simulink library "Memory_Blocks_Lib"  (R2023a)
settings: Solver=ode45  StartTime=0.0  StopTime=10.0  RelTol=1e-3  EnableMultiTasking=on
libraries: simulink_extras x17
settings Model: Creator=uzivatel  LastModifiedBy=Jozko Mrkvicka
settings SolverCC: AlgebraicLoopSolver=TrustRegion
settings DataIOCC: LimitDataPoints=on  SaveFormat=Array  ReturnWorkspaceOutputs=off
settings OptimizationCC: LifeSpan=inf
settings DebuggingCC: UnderspecifiedInitializationDetection=Classic  MergeDetectMultiDrivingBlocksExec=none  SolverPrmCheckMsg=warning  UnconnectedInputMsg=warning  UnconnectedOutputMsg=warning  UnconnectedLineMsg=warning  StateNameClashWarn=warning  SFUnexpectedBacktrackingDiag=warning  SFNoUnconditionalDefaultTransitionDiag=warning  ArithmeticOperatorsInVariantConditions=warning
settings HardwareCC: ProdBitPerPointer=32  ProdBitPerSizeT=32  ProdBitPerPtrDiffT=32  ProdLargestAtomicFloat=None  ProdIntDivRoundTo=Undefined  ProdEndianess=Unspecified  ProdWordSize=32  ProdHWDeviceType=32-bit Generic
settings ModelReferenceCC: EnableRefExpFcnMdlSchedulingChecks=on  PropagateSignalLabelsOutOfModel=off
settings SFSimCC: SimUseLocalCustomCode=off  CustomCodeUndefinedFunction=UseInterfaceOnly
settings RTWCC: RTWUseLocalCustomCode=off
settings CodeAppCC: StateflowObjectComments=on
settings GRTTargetCC: TargetLangStandard=C89/C90 (ANSI)
settings ConfigComp: CovMetricSettings=dw  CovSaveCumulativeToWorkspaceVar=on  CovSaveSingleToWorkspaceVar=on  CovExternalEMLEnable=off

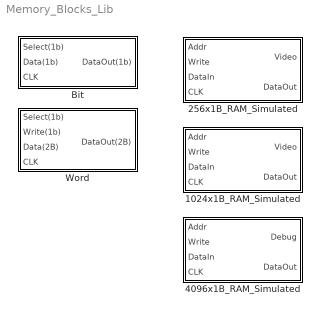
== system Memory_Blocks_Lib ==
  1024x1B_RAM_Simulated : MATLAB Function  TreatAsAtomicUnit=on
  256x1B_RAM_Simulated : MATLAB Function  TreatAsAtomicUnit=on
  4096x1B_RAM_Simulated : MATLAB Function  TreatAsAtomicUnit=on
  Bit : Subsystem
  Word : Subsystem

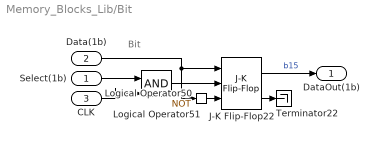
== system Memory_Blocks_Lib/Bit ==
  note: Bit
  Select(1b) : Inport  OutDataTypeStr=boolean
  Data(1b) : Inport  Port=2  OutDataTypeStr=boolean
  CLK : Inport  Port=3  OutDataTypeStr=double
  J-K Flip-Flop22 : simulink_extras/Flip Flops/J-K Flip-Flop  initial_condition=0
  Logical Operator50 : Logic  Operator=NOT  IconShape=distinctive  AllPortsSameDT=off  OutDataTypeStr=boolean
  Logical Operator51 : Logic  IconShape=distinctive  AllPortsSameDT=off  OutDataTypeStr=boolean
  Terminator22 : Terminator
  DataOut(1b) : Outport
  wires:
  Select(1b)/1 -> Logical Operator51/1
  Logical Operator50/1 -> J-K Flip-Flop22/3
  CLK/1 -> Logical Operator51/2
  Data(1b)/1 -> Logical Operator50/1, J-K Flip-Flop22/1
  J-K Flip-Flop22/2 -> Terminator22/1
  J-K Flip-Flop22/1 -> DataOut(1b)/1  "b15"
  Logical Operator51/1 -> J-K Flip-Flop22/2

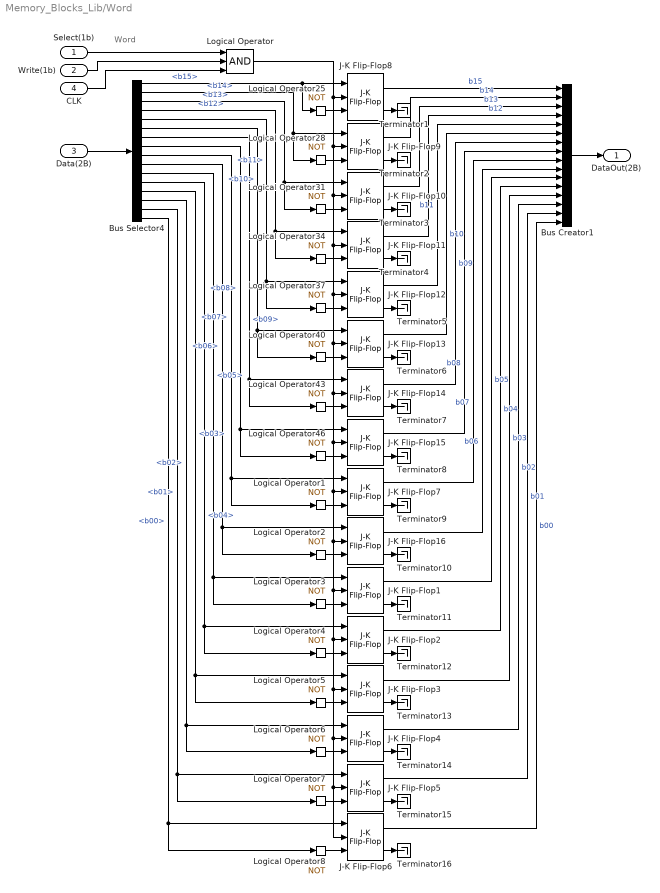
== system Memory_Blocks_Lib/Word ==
  note: Word
  Select(1b) : Inport
  Write(1b) : Inport  Port=2
  Data(2B) : Inport  Port=3
  CLK : Inport  Port=4
  Bus Creator1 : BusCreator  Inputs=16
  Bus Selector4 : BusSelector  OutputSignals=b15,b14,b13,b12,b11,b10,b09,b08,b07,b06,b05,b04,b03,b02,b01,b00
  J-K Flip-Flop{1..16} (16 alike) : simulink_extras/Flip Flops/J-K Flip-Flop  initial_condition=0
  Logical Operator : Logic  Inputs=3  IconShape=distinctive  AllPortsSameDT=off  OutDataTypeStr=boolean
  Logical Operator{1..8,25,28,31,34,37,40,43,46} (16 alike) : Logic  Operator=NOT  IconShape=distinctive  AllPortsSameDT=off  OutDataTypeStr=boolean
  Terminator{1..16} (16 alike) : Terminator
  DataOut(2B) : Outport
  wires:
  Write(1b)/1 -> Logical Operator/2
  Data(2B)/1 -> Bus Selector4/1
  Logical Operator25/1 -> J-K Flip-Flop8/3
  J-K Flip-Flop8/1 -> Bus Creator1/1  "b15"
  J-K Flip-Flop8/2 -> Terminator1/1
  Logical Operator28/1 -> J-K Flip-Flop9/3
  J-K Flip-Flop9/1 -> Bus Creator1/2  "b14"
  J-K Flip-Flop9/2 -> Terminator2/1
  Bus Selector4/2 -> Logical Operator28/1, J-K Flip-Flop9/1  "<b14>"
  Logical Operator31/1 -> J-K Flip-Flop10/3
  J-K Flip-Flop10/1 -> Bus Creator1/3  "b13"
  J-K Flip-Flop10/2 -> Terminator3/1
  Bus Selector4/3 -> Logical Operator31/1, J-K Flip-Flop10/1  "<b13>"
  Logical Operator34/1 -> J-K Flip-Flop11/3
  J-K Flip-Flop11/1 -> Bus Creator1/4  "b12"
  J-K Flip-Flop11/2 -> Terminator4/1
  Bus Selector4/4 -> J-K Flip-Flop11/1, Logical Operator34/1  "<b12>"
  Logical Operator37/1 -> J-K Flip-Flop12/3
  J-K Flip-Flop12/1 -> Bus Creator1/5  "b11"
  J-K Flip-Flop12/2 -> Terminator5/1
  Bus Selector4/5 -> J-K Flip-Flop12/1, Logical Operator37/1  "<b11>"
  Logical Operator40/1 -> J-K Flip-Flop13/3
  J-K Flip-Flop13/1 -> Bus Creator1/6  "b10"
  J-K Flip-Flop13/2 -> Terminator6/1
  Bus Selector4/6 -> J-K Flip-Flop13/1, Logical Operator40/1  "<b10>"
  Logical Operator43/1 -> J-K Flip-Flop14/3
  J-K Flip-Flop14/1 -> Bus Creator1/7  "b09"
  J-K Flip-Flop14/2 -> Terminator7/1
  Bus Selector4/7 -> J-K Flip-Flop14/1, Logical Operator43/1  "<b09>"
  Logical Operator46/1 -> J-K Flip-Flop15/3
  J-K Flip-Flop15/1 -> Bus Creator1/8  "b08"
  J-K Flip-Flop15/2 -> Terminator8/1
  Bus Selector4/8 -> J-K Flip-Flop15/1, Logical Operator46/1  "<b08>"
  Bus Selector4/1 -> Logical Operator25/1, J-K Flip-Flop8/1  "<b15>"
  CLK/1 -> Logical Operator/3
  Select(1b)/1 -> Logical Operator/1
  J-K Flip-Flop5/2 -> Terminator15/1
  Bus Selector4/14 -> Logical Operator6/1, J-K Flip-Flop4/1  "<b02>"
  J-K Flip-Flop16/2 -> Terminator10/1
  Logical Operator1/1 -> J-K Flip-Flop7/3
  Logical Operator5/1 -> J-K Flip-Flop3/3
  Logical Operator/1 -> J-K Flip-Flop6/2, J-K Flip-Flop5/2, J-K Flip-Flop4/2, J-K Flip-Flop3/2, J-K Flip-Flop2/2, J-K Flip-Flop1/2, J-K Flip-Flop16/2, J-K Flip-Flop7/2, J-K Flip-Flop15/2, J-K Flip-Flop14/2, J-K Flip-Flop13/2, J-K Flip-Flop12/2, J-K Flip-Flop11/2, J-K Flip-Flop10/2, J-K Flip-Flop9/2, J-K Flip-Flop8/2
  J-K Flip-Flop6/1 -> Bus Creator1/16  "b00"
  J-K Flip-Flop5/1 -> Bus Creator1/15  "b01"
  J-K Flip-Flop6/2 -> Terminator16/1
  J-K Flip-Flop4/2 -> Terminator14/1
  Bus Selector4/15 -> J-K Flip-Flop5/1, Logical Operator7/1  "<b01>"
  Logical Operator7/1 -> J-K Flip-Flop5/3
  Bus Selector4/10 -> J-K Flip-Flop16/1, Logical Operator2/1  "<b06>"
  J-K Flip-Flop4/1 -> Bus Creator1/14  "b02"
  J-K Flip-Flop16/1 -> Bus Creator1/10  "b06"
  Logical Operator8/1 -> J-K Flip-Flop6/3
  J-K Flip-Flop3/2 -> Terminator13/1
  Logical Operator4/1 -> J-K Flip-Flop2/3
  Bus Selector4/13 -> J-K Flip-Flop3/1, Logical Operator5/1  "<b03>"
  J-K Flip-Flop2/1 -> Bus Creator1/12  "b04"
  Logical Operator6/1 -> J-K Flip-Flop4/3
  J-K Flip-Flop3/1 -> Bus Creator1/13  "b03"
  Logical Operator2/1 -> J-K Flip-Flop16/3
  J-K Flip-Flop1/2 -> Terminator11/1
  J-K Flip-Flop1/1 -> Bus Creator1/11  "b05"
  Bus Selector4/11 -> J-K Flip-Flop1/1, Logical Operator3/1  "<b05>"
  Bus Selector4/16 -> J-K Flip-Flop6/1, Logical Operator8/1  "<b00>"
  Logical Operator3/1 -> J-K Flip-Flop1/3
  J-K Flip-Flop2/2 -> Terminator12/1
  J-K Flip-Flop7/1 -> Bus Creator1/9  "b07"
  Bus Selector4/9 -> J-K Flip-Flop7/1, Logical Operator1/1  "<b07>"
  J-K Flip-Flop7/2 -> Terminator9/1
  Bus Selector4/12 -> J-K Flip-Flop2/1, Logical Operator4/1  "<b04>"
  Bus Creator1/1 -> DataOut(2B)/1

== matlab function Memory_Blocks_Lib/4096x1B_RAM_Simulated ==
  data: Addr input Bus: BUS_UINT16_T; Write input; Debug output; DataIn input Bus: BUS_UINT16_T size=1; CLK input; DataOut output Bus: BUS_UINT16_T
function [Debug, DataOut] = RAM(Addr, Write, DataIn, CLK)
    persistent ram_memory;

    if (isempty(ram_memory))
        ram_memory = zeros(1, 4096, 'uint8');
    end

    %Convert the DataIn parameter to uint8.
    temp =                       ...
        128 * DataIn.b07 +  ...
        64  * DataIn.b06 +  ...
        32  * DataIn.b05 +  ...
        16  * DataIn.b04 +  ...
        8   * DataIn.b03 +  ...
        4   * DataIn.b02 +  ...
        2   * DataIn.b01 +  ...
        1   * DataIn.b00;
    data = uint8(temp);

    %Convert the Addr parameter to uint16.
    temp =                      ...
        2048 * Addr.b11  +  ...
        1024 * Addr.b10  +  ...
        512  * Addr.b09  +  ...
        256  * Addr.b08  +  ...
        128  * Addr.b07 +  ...
        64   * Addr.b06 +  ...
        32   * Addr.b05 +  ...
        16   * Addr.b04 +  ...
        8    * Addr.b03 +  ...
        4    * Addr.b02 +  ...
        2    * Addr.b01 +  ...
        1    * Addr.b00;
    address = uint16(temp);

    if ((true == Write) && (1 == CLK))
        ram_memory(1, address + 1) = data;
    end

    %Convert the DataOut parameter to BUS_UINT16_T.
    temp = ram_memory(1, address + 1);
    temp = dec2bin(temp, 8);
    DataOut.b15 = false;
    DataOut.b14 = false;
    DataOut.b13 = false;
    DataOut.b12 = false;
    DataOut.b11 = false;
    DataOut.b10 = false;
    DataOut.b09 = false;
    DataOut.b08 = false;
    if (1 == (temp(1) - 48)) DataOut.b07 = true; else DataOut.b07 = false; end
    if (1 == (temp(2) - 48)) DataOut.b06 = true; else DataOut.b06 = false; end
    if (1 == (temp(3) - 48)) DataOut.b05 = true; else DataOut.b05 = false; end
    if (1 == (temp(4) - 48)) DataOut.b04 = true; else DataOut.b04 = false; end
    if (1 == (temp(5) - 48)) DataOut.b03 = true; else DataOut.b03 = false; end
    if (1 == (temp(6) - 48)) DataOut.b02 = true; else DataOut.b02 = false; end
    if (1 == (temp(7) - 48)) DataOut.b01 = true; else DataOut.b01 = false; end
    if (1 == (temp(8) - 48)) DataOut.b00 = true; else DataOut.b00 = false; end

    Debug = ram_memory;    
end

== matlab function Memory_Blocks_Lib/256x1B_RAM_Simulated ==
  data: Addr input Bus: BUS_UINT16_T; Write input; Video output; DataIn input Bus: BUS_UINT16_T size=1; CLK input; DataOut output Bus: BUS_UINT16_T
function [Video, DataOut] = RAM(Addr, Write, DataIn, CLK)
    persistent ram_memory;

    if (isempty(ram_memory))
        ram_memory = zeros(1, 256, 'uint8');
    end

    %Convert the DataIn parameter to uint8.
    temp =                       ...
        128 * DataIn.signal9  +  ...
        64  * DataIn.signal10 +  ...
        32  * DataIn.signal11 +  ...
        16  * DataIn.signal12 +  ...
        8   * DataIn.signal13 +  ...
        4   * DataIn.signal14 +  ...
        2   * DataIn.signal15 +  ...
        1   * DataIn.signal16;
    data = uint8(temp);

    %Convert the Addr parameter to uint16.
    temp =                     ...
        128 * Addr.signal9  +  ...
        64  * Addr.signal10 +  ...
        32  * Addr.signal11 +  ...
        16  * Addr.signal12 +  ...
        8   * Addr.signal13 +  ...
        4   * Addr.signal14 +  ...
        2   * Addr.signal15 +  ...
        1   * Addr.signal16;
    address = uint16(temp);

    if ((true == Write) && (1 == CLK))
        ram_memory(1, address + 1) = data;
    end

    %Convert the DataOut parameter to BUS_UINT16_T.
    temp = ram_memory(1, address + 1);
    temp = dec2bin(temp, 8);
    DataOut.signal1 = false;
    DataOut.signal2 = false;
    DataOut.signal3 = false;
    DataOut.signal4 = false;
    DataOut.signal5 = false;
    DataOut.signal6 = false;
    DataOut.signal7 = false;
    DataOut.signal8 = false;
    if (1 == (temp(1) - 48)) DataOut.signal9  = true; else DataOut.signal9  = false; end
    if (1 == (temp(2) - 48)) DataOut.signal10 = true; else DataOut.signal10 = false; end
    if (1 == (temp(3) - 48)) DataOut.signal11 = true; else DataOut.signal11 = false; end
    if (1 == (temp(4) - 48)) DataOut.signal12 = true; else DataOut.signal12 = false; end
    if (1 == (temp(5) - 48)) DataOut.signal13 = true; else DataOut.signal13 = false; end
    if (1 == (temp(6) - 48)) DataOut.signal14 = true; else DataOut.signal14 = false; end
    if (1 == (temp(7) - 48)) DataOut.signal15 = true; else DataOut.signal15 = false; end
    if (1 == (temp(8) - 48)) DataOut.signal16 = true; else DataOut.signal16 = false; end

    Video = ram_memory;    
end

== matlab function Memory_Blocks_Lib/1024x1B_RAM_Simulated ==
  data: Addr input Bus: BUS_UINT16_T; Write input; Video output; DataIn input Bus: BUS_UINT16_T size=1; CLK input; DataOut output Bus: BUS_UINT16_T
function [Video, DataOut] = RAM(Addr, Write, DataIn, CLK)
    persistent ram_memory;

    if (isempty(ram_memory))
        % ram_memory = zeros(1, 1024, 'uint8');
        ram_memory = zeros(1024, 1, 'uint8');
    end

    %Convert the DataIn parameter to uint8.
    temp =                       ...
        128 * DataIn.b07 +  ...
        64  * DataIn.b06 +  ...
        32  * DataIn.b05 +  ...
        16  * DataIn.b04 +  ...
        8   * DataIn.b03 +  ...
        4   * DataIn.b02 +  ...
        2   * DataIn.b01 +  ...
        1   * DataIn.b00;
    data = uint8(temp);

    %Convert the Addr parameter to uint16.
    temp =                      ...
        512  * Addr.b09 +  ...
        256  * Addr.b08 +  ...
        128  * Addr.b07 +  ...
        64   * Addr.b06 +  ...
        32   * Addr.b05 +  ...
        16   * Addr.b04 +  ...
        8    * Addr.b03 +  ...
        4    * Addr.b02 +  ...
        2    * Addr.b01 +  ...
        1    * Addr.b00;
    address = uint16(temp);

    if ((true == Write) && (1 == CLK))
        % ram_memory(1, address + 1) = data;
        ram_memory(address + 1, 1) = data;
    end

    %Convert the DataOut parameter to BUS_UINT16_T.
    % temp = ram_memory(1, address + 1);
    temp = ram_memory(address + 1, 1);
    temp = dec2bin(temp, 8);
    DataOut.b15 = false;
    DataOut.b14 = false;
    DataOut.b13 = false;
    DataOut.b12 = false;
    DataOut.b11 = false;
    DataOut.b10 = false;
    DataOut.b09 = false;
    DataOut.b08 = false;
    if (1 == (temp(1) - 48)) DataOut.b07 = true; else DataOut.b07 = false; end
    if (1 == (temp(2) - 48)) DataOut.b06 = true; else DataOut.b06 = false; end
    if (1 == (temp(3) - 48)) DataOut.b05 = true; else DataOut.b05 = false; end
    if (1 == (temp(4) - 48)) DataOut.b04 = true; else DataOut.b04 = false; end
    if (1 == (temp(5) - 48)) DataOut.b03 = true; else DataOut.b03 = false; end
    if (1 == (temp(6) - 48)) DataOut.b02 = true; else DataOut.b02 = false; end
    if (1 == (temp(7) - 48)) DataOut.b01 = true; else DataOut.b01 = false; end
    if (1 == (temp(8) - 48)) DataOut.b00 = true; else DataOut.b00 = false; end

    Video = ram_memory;    
end
